simulink model "Target_Control_System"  (R2021b)
settings: Solver=FixedStepDiscrete  StartTime=0.0  StopTime=5  RelTol=1e-3
PreLoadFcn:
  | RTWConfigurationCB('preloadfcn', bdroot);
PostLoadFcn:
  | load('configuration/data_struct.mat');
  | load('configuration/fluxMaps_propMotor.mat');
  | load('configuration/parameterInit_PROP.mat');
  | load('configuration/parameterInit_PUMP.mat');
  | load('configuration/parameterInit_PITCH.mat');
  | load('configuration/parameterInit_TILT.mat');
  | %load('configuration/base_workspace_signal_definition.mat');
  | %load('resolvedatastores_to_baseworkspace_for_faster_simulation.mat');
model workspace (MAT data in the model file):
  SIMULATION_OPTIONS : Simulink.Parameter (value not decoded)
  TARGET_CODE_GEN : Simulink.Parameter (value not decoded)
  TCS_SAMPLE_FREQ_HZ : Simulink.Parameter (value not decoded)
symbols that are objects in the model workspace (value not decoded): TARGET_CODE_GEN, TCS_SAMPLE_FREQ_HZ
undefined symbols (not defined in the file): A_DQ_REF_LPF_INIT__PITCH, A_DQ_REF_LPF_INIT__PROP, A_DQ_REF_LPF_INIT__PUMP, A_DQ_REF_LPF_INIT__TILT, A_OBSERVER_CONFIDENCE_INIT__PITCH, A_OBSERVER_CONFIDENCE_INIT__PROP, A_OBSERVER_CONFIDENCE_INIT__PUMP, A_OBSERVER_CONFIDENCE_INIT__TILT, ACTUATOR_MAX_ANGLE_TRIP__PITCH, ACTUATOR_MIN_ANGLE_TRIP__PITCH, ACTUATOR_POS_SENSOR_INV_DIRECTION__PITCH, ACTUATOR_POS_SENSOR_INV_DIRECTION__TILT, ACTUATOR_POS_SENSOR_OFFSET__PITCH, ACTUATOR_POS_SENSOR_OFFSET__TILT, ADC_scaler1_baseaddr_TILT, ADC_SCALER_FLOAT_TO_FIXPOINT_EXPANSION, ANGLE_ELEC_FROM_SENSOR_OFFSET_INIT__PITCH, ANGLE_ELEC_FROM_SENSOR_OFFSET_INIT__PROP, ANGLE_ELEC_FROM_SENSOR_OFFSET_INIT__PUMP, ANGLE_ELEC_FROM_SENSOR_OFFSET_INIT__TILT, AUTO_CLEAR_FAULTS_ENABLED__PITCH, AUTO_CLEAR_FAULTS_ENABLED__PROP, AUTO_CLEAR_FAULTS_ENABLED__PUMP, AUTO_CLEAR_FAULTS_ENABLED__TILT, AUTO_CLEAR_FAULTS_WAIT_TICKS__PITCH, AUTO_CLEAR_FAULTS_WAIT_TICKS__PROP, AUTO_CLEAR_FAULTS_WAIT_TICKS__PUMP, AUTO_CLEAR_FAULTS_WAIT_TICKS__TILT, AUTO_I_ZERO_IDLE_TICKS__PITCH, AUTO_I_ZERO_IDLE_TICKS__PROP, AUTO_I_ZERO_IDLE_TICKS__PUMP, AUTO_I_ZERO_IDLE_TICKS__TILT, AUTO_I_ZERO_OFFSET_IDC_THRESHOLD__PITCH, AUTO_I_ZERO_OFFSET_IDC_THRESHOLD__PROP, AUTO_I_ZERO_OFFSET_IDC_THRESHOLD__PUMP, AUTO_I_ZERO_OFFSET_IDC_THRESHOLD__TILT, AUTO_I_ZERO_OFFSET_IPH_THRESHOLD__PITCH, AUTO_I_ZERO_OFFSET_IPH_THRESHOLD__PROP, AUTO_I_ZERO_OFFSET_IPH_THRESHOLD__PUMP, AUTO_I_ZERO_OFFSET_IPH_THRESHOLD__TILT, AUTO_SENSORLESS_SWITCHOVER_DISABLE_OMEGA, AUTO_SENSORLESS_SWITCHOVER_ENABLE_OMEGA, AUTO_SENSORLESS_SWITCHOVER_MIN_CONFIDENCE, AUXILIARY_PROTECTION_UNIT_BASEADDR__TILT, blanking_max_error_omega_INIT_PITCH, blanking_max_error_omega_INIT_TILT, blanking_max_error_position_INIT_PITCH, blanking_max_error_position_INIT_TILT, BRUTE_START_I_Q_REF_RAMP_SPEED__PITCH, BRUTE_START_I_Q_REF_RAMP_SPEED__PROP, BRUTE_START_I_Q_REF_RAMP_SPEED__PUMP, BRUTE_START_I_Q_REF_RAMP_SPEED__TILT, CONTROL_LOOP_DT_INIT__PITCH, CONTROL_LOOP_DT_INIT__PROP, CONTROL_LOOP_DT_INIT__PUMP, CONTROL_LOOP_DT_INIT__TILT, CORRECTION_FILTER_SCALE__PITCH, CORRECTION_FILTER_SCALE__PROP, CORRECTION_FILTER_SCALE__PUMP, CORRECTION_FILTER_SCALE__TILT ... (+458)
libraries: simulink x178, Reusables_Lib x24
(part 34 of 47)

== system Target_Control_System/Target_Control_System/MainLoop/pumpMotor_mainLoop/motorTaskMainFastStep(&oPump)/Control Loops - Pump/Sim Options Pump OmegaERef Variant Subsystem/Sim Options 1 Pump OmegaE Subsystem ==
  Constant : Constant  Value=2000  OutDataTypeStr=single  SampleTime=-1
  Constant1 : Constant  Value=0  OutDataTypeStr=uint32  SampleTime=-1
  Data Store Write : DataStoreWrite  DataStoreName=oPump  DataStoreElements=oPump.oMot_.oState_.oRampDataOmegaERef_.fSetpoint_  IndexOptions=Index vector (dialog)  Indices=1  OutputSizes=1
  Data Store Write1 : DataStoreWrite  DataStoreName=oPump  DataStoreElements=oPump.oMot_.oState_.uiSpeedControllerActive_  IndexOptions=Index vector (dialog)  Indices=1  OutputSizes=1
  Out1 : Outport
  wires:
  Constant1/1 -> Data Store Write1/1
  Constant/1 -> Data Store Write/1, Out1/1

== system Target_Control_System/Target_Control_System/MainLoop/pumpMotor_mainLoop/motorTaskMainFastStep(&oPump)/Control Loops - Pump/Subsystem/Set Iq Ref Pump ==
  fIqRefFromSpeedController : Inport
  Enable : EnablePort
  Data Store Read : DataStoreRead  DataStoreName=oPitch  DataStoreElements=oPitch.oMot_.oState_.oFilterDataForSpeedControlIqRef_.afConstantsA_.h0  IndexOptions=Index vector (dialog)  Indices=1  OutputSizes=1
  Data Store Read1 : DataStoreRead  DataStoreName=oPitch  DataStoreElements=oPitch.oMot_.oState_.oFilterDataForSpeedControlIqRef_.afConstantsA_.h1  IndexOptions=Index vector (dialog)  Indices=1  OutputSizes=1
  Data Store Read2 : DataStoreRead  DataStoreName=oPitch  DataStoreElements=oPitch.oMot_.oState_.oFilterDataForSpeedControlIqRef_.afConstantsA_.h2  IndexOptions=Index vector (dialog)  Indices=1  OutputSizes=1
  Data Store Read3 : DataStoreRead  DataStoreName=oPitch  DataStoreElements=oPitch.oMot_.oState_.oFilterDataForSpeedControlIqRef_.afConstantsB_.h0  IndexOptions=Index vector (dialog)  Indices=1  OutputSizes=1
  Data Store Read4 : DataStoreRead  DataStoreName=oPitch  DataStoreElements=oPitch.oMot_.oState_.oFilterDataForSpeedControlIqRef_.afConstantsB_.h1  IndexOptions=Index vector (dialog)  Indices=1  OutputSizes=1
  Data Store Read5 : DataStoreRead  DataStoreName=oPitch  DataStoreElements=oPitch.oMot_.oState_.oFilterDataForSpeedControlIqRef_.afConstantsB_.h2  IndexOptions=Index vector (dialog)  Indices=1  OutputSizes=1
  Data Store Read6 : DataStoreRead  DataStoreName=oPitch  DataStoreElements=oPitch.oMot_.oState_.oFilterDataForSpeedControlIqRef_.afPreviousInputs_.h0  IndexOptions=Index vector (dialog)  Indices=1  OutputSizes=1
  Data Store Read7 : DataStoreRead  DataStoreName=oPitch  DataStoreElements=oPitch.oMot_.oState_.oFilterDataForSpeedControlIqRef_.afPreviousInputs_.h1  IndexOptions=Index vector (dialog)  Indices=1  OutputSizes=1
  Data Store Read8 : DataStoreRead  DataStoreName=oPitch  DataStoreElements=oPitch.oMot_.oState_.oFilterDataForSpeedControlIqRef_.afPreviousOutputs_.h0  IndexOptions=Index vector (dialog)  Indices=1  OutputSizes=1
  Data Store Read9 : DataStoreRead  DataStoreName=oPitch  DataStoreElements=oPitch.oMot_.oState_.oFilterDataForSpeedControlIqRef_.afPreviousOutputs_.h1  IndexOptions=Index vector (dialog)  Indices=1  OutputSizes=1
  Data Store Write1 : DataStoreWrite  DataStoreName=oPitch  DataStoreElements=oPitch.oMot_.oState_.oFilterDataForSpeedControlIqRef_.fFilterOutput_  IndexOptions=Index vector (dialog)  Indices=1  OutputSizes=1
  Data Store Write2 : DataStoreWrite  DataStoreName=oPitch  DataStoreElements=oPitch.oMot_.oState_.oFilterDataForSpeedControlIqRef_.afPreviousOutputs_.h0  IndexOptions=Index vector (dialog)  Indices=1  OutputSizes=1
  Data Store Write3 : DataStoreWrite  DataStoreName=oPitch  DataStoreElements=oPitch.oMot_.oState_.oFilterDataForSpeedControlIqRef_.afPreviousOutputs_.h1  IndexOptions=Index vector (dialog)  Indices=1  OutputSizes=1
  Data Store Write4 : DataStoreWrite  DataStoreName=oPitch  DataStoreElements=oPitch.oMot_.oState_.oFilterDataForSpeedControlIqRef_.afPreviousInputs_.h0  IndexOptions=Index vector (dialog)  Indices=1  OutputSizes=1
  Data Store Write5 : DataStoreWrite  DataStoreName=oPitch  DataStoreElements=oPitch.oMot_.oState_.oFilterDataForSpeedControlIqRef_.afPreviousInputs_.h1  IndexOptions=Index vector (dialog)  Indices=1  OutputSizes=1
  softwareIirFilterStep() : Subsystem
  fIqRefBeforeRamp : Outport
  wires:
  softwareIirFilterStep()/1(*afPreviousInputs1) -> Data Store Write5/1
  softwareIirFilterStep()/2(*afPreviousInputs0) -> Data Store Write4/1
  softwareIirFilterStep()/3(*afPreviousOutputs1) -> Data Store Write3/1
  softwareIirFilterStep()/4(*afPreviousOutputs0) -> Data Store Write2/1
  softwareIirFilterStep()/5(fFilterOutput) -> Data Store Write1/1
  Data Store Read6/1 -> softwareIirFilterStep()/8(afPreviousInputs0)
  Data Store Read7/1 -> softwareIirFilterStep()/9(afPreviousInputs1)
  Data Store Read8/1 -> softwareIirFilterStep()/10(afPreviousOutputs0)
  Data Store Read9/1 -> softwareIirFilterStep()/11(afPreviousOutputs1)
  Data Store Read2/1 -> softwareIirFilterStep()/7(afConstantsA2)
  Data Store Read1/1 -> softwareIirFilterStep()/6(afConstantsA1)
  Data Store Read/1 -> softwareIirFilterStep()/5(afConstantsA0)
  Data Store Read3/1 -> softwareIirFilterStep()/2(afConstantsB0)
  Data Store Read4/1 -> softwareIirFilterStep()/3(afConstantsB1)
  Data Store Read5/1 -> softwareIirFilterStep()/4(afConstantsB2)
  fIqRefFromSpeedController/1 -> softwareIirFilterStep()/1(newInput), fIqRefBeforeRamp/1

== system Target_Control_System/Target_Control_System/MainLoop/pumpMotor_mainLoop/motorTaskMainFastStep(&oPump)/Control Loops - Pump/Subsystem/piControllerStep(&oPiDataRpm_) ==
  fActual : Inport
  fTarget : Inport  Port=2
  fScale : Inport  Port=3
  Enable : EnablePort
  Data Store Read62 : DataStoreRead  DataStoreName=oPump  DataStoreElements=oPump.oMot_.oParam_.oPiDataRpm_.oParameter_.fOutMin_  IndexOptions=Index vector (dialog)  Indices=1  OutputSizes=1
  Data Store Read81 : DataStoreRead  DataStoreName=oPump  DataStoreElements=oPump.oMot_.oParam_.oPiDataRpm_.oParameter_.fKp_  IndexOptions=Index vector (dialog)  Indices=1  OutputSizes=1
  Data Store Read85 : DataStoreRead  DataStoreName=oPump  DataStoreElements=oPump.oMot_.oParam_.oPiDataRpm_.fState_  IndexOptions=Index vector (dialog)  Indices=1  OutputSizes=1
  Data Store Read86 : DataStoreRead  DataStoreName=oPump  DataStoreElements=oPump.oMot_.oParam_.oPiDataRpm_.oParameter_.fLoopDt_  IndexOptions=Index vector (dialog)  Indices=1  OutputSizes=1
  Data Store Read88 : DataStoreRead  DataStoreName=oPump  DataStoreElements=oPump.oMot_.oParam_.oPiDataRpm_.oParameter_.fIntMax_  IndexOptions=Index vector (dialog)  Indices=1  OutputSizes=1
  Data Store Read89 : DataStoreRead  DataStoreName=oPump  DataStoreElements=oPump.oMot_.oParam_.oPiDataRpm_.oParameter_.fOutMax_  IndexOptions=Index vector (dialog)  Indices=1  OutputSizes=1
  Data Store Read90 : DataStoreRead  DataStoreName=oPump  DataStoreElements=oPump.oMot_.oParam_.oPiDataRpm_.oParameter_.fIntMin_  IndexOptions=Index vector (dialog)  Indices=1  OutputSizes=1
  Data Store Read91 : DataStoreRead  DataStoreName=oPump  DataStoreElements=oPump.oMot_.oParam_.oPiDataRpm_.oParameter_.fKi_  IndexOptions=Index vector (dialog)  Indices=1  OutputSizes=1
  Data Store Write21 : DataStoreWrite  DataStoreName=oPump  DataStoreElements=oPump.oMot_.oParam_.oPiDataRpm_.fState_  IndexOptions=Index vector (dialog)  Indices=1  OutputSizes=1
  oPiDataRpm_ : Subsystem
  fOutput : Outport
  wires:
  Data Store Read62/1 -> oPiDataRpm_/10(fOutMin)
  fActual/1 -> oPiDataRpm_/1(fActual)
  fScale/1 -> oPiDataRpm_/5(fScale)
  Data Store Read88/1 -> oPiDataRpm_/7(fIntMax)
  Data Store Read86/1 -> oPiDataRpm_/6(fLoopDt)
  oPiDataRpm_/2(*fpState) -> Data Store Write21/1
  oPiDataRpm_/1(fOutput) -> fOutput/1
  fTarget/1 -> oPiDataRpm_/2(fTarget)
  Data Store Read91/1 -> oPiDataRpm_/4(fKi)
  Data Store Read89/1 -> oPiDataRpm_/8(fOutMax)
  Data Store Read90/1 -> oPiDataRpm_/9(fIntMin)
  Data Store Read85/1 -> oPiDataRpm_/11(fState)
  Data Store Read81/1 -> oPiDataRpm_/3(fKp)

== system Target_Control_System/Target_Control_System/MainLoop/pumpMotor_mainLoop/motorTaskMainFastStep(&oPump)/Control Loops - Pump/Subsystem/pid2ControllerStep(&oPid2DataRpmCtrl_) ==
  fState : Inport
  fActual : Inport  Port=2
  fTarget : Inport  Port=3
  fActualDdt : Inport  Port=4
  Enable : EnablePort
  Data Store Read1 : DataStoreRead  DataStoreName=oPump  DataStoreElements=oPump.oMot_.oParam_.oPid2DataRpmCtrl_.oParameter_.fKi_  IndexOptions=Index vector (dialog)  Indices=1  OutputSizes=1
  Data Store Read10 : DataStoreRead  DataStoreName=oPump  DataStoreElements=oPump.oMot_.oParam_.oPid2DataRpmCtrl_.oParameter_.ipInhibitTarget_  IndexOptions=Index vector (dialog)  Indices=1  OutputSizes=1
  Data Store Read11 : DataStoreRead  DataStoreName=oPump  DataStoreElements=oPump.oMot_.oParam_.oPid2DataRpmCtrl_.oParameter_.fBlankingMaxError_  IndexOptions=Index vector (dialog)  Indices=1  OutputSizes=1
  Data Store Read12 : DataStoreRead  DataStoreName=oPump  DataStoreElements=oPump.oMot_.oParam_.oPid2DataRpmCtrl_.oParameter_.fLargeErrorThresholdNegative_  IndexOptions=Index vector (dialog)  Indices=1  OutputSizes=1
  Data Store Read13 : DataStoreRead  DataStoreName=oPump  DataStoreElements=oPump.oMot_.oParam_.oPid2DataRpmCtrl_.oParameter_.fLargeErrorThresholdPositive_  IndexOptions=Index vector (dialog)  Indices=1  OutputSizes=1
  Data Store Read14 : DataStoreRead  DataStoreName=oPump  DataStoreElements=oPump.oMot_.oParam_.oPid2DataRpmCtrl_.oParameter_.fIntegratorLeakFactor_  IndexOptions=Index vector (dialog)  Indices=1  OutputSizes=1
  Data Store Read15 : DataStoreRead  DataStoreName=oPump  DataStoreElements=oPump.oMot_.oParam_.oPid2DataRpmCtrl_.oParameter_.fErrorReduction_  IndexOptions=Index vector (dialog)  Indices=1  OutputSizes=1
  Data Store Read2 : DataStoreRead  DataStoreName=oPump  DataStoreElements=oPump.oMot_.oParam_.oPid2DataRpmCtrl_.oParameter_.fKd_  IndexOptions=Index vector (dialog)  Indices=1  OutputSizes=1
  Data Store Read20 : DataStoreRead  DataStoreName=oPump  DataStoreElements=oPump.oMot_.oParam_.oPid2DataRpmCtrl_.oParameter_.fKp_  IndexOptions=Index vector (dialog)  Indices=1  OutputSizes=1
  Data Store Read3 : DataStoreRead  DataStoreName=oPump  DataStoreElements=oPump.oMot_.oParam_.oPid2DataRpmCtrl_.oParameter_.fIntMin_  IndexOptions=Index vector (dialog)  Indices=1  OutputSizes=1
  Data Store Read4 : DataStoreRead  DataStoreName=oPump  DataStoreElements=oPump.oMot_.oParam_.oPid2DataRpmCtrl_.oParameter_.fIntMax_  IndexOptions=Index vector (dialog)  Indices=1  OutputSizes=1
  Data Store Read5 : DataStoreRead  DataStoreName=oPump  DataStoreElements=oPump.oMot_.oParam_.oPid2DataRpmCtrl_.oParameter_.fDMin_  IndexOptions=Index vector (dialog)  Indices=1  OutputSizes=1
  Data Store Read6 : DataStoreRead  DataStoreName=oPump  DataStoreElements=oPump.oMot_.oParam_.oPid2DataRpmCtrl_.oParameter_.fDMax_  IndexOptions=Index vector (dialog)  Indices=1  OutputSizes=1
  Data Store Read7 : DataStoreRead  DataStoreName=oPump  DataStoreElements=oPump.oMot_.oParam_.oPid2DataRpmCtrl_.oParameter_.fOutMin_  IndexOptions=Index vector (dialog)  Indices=1  OutputSizes=1
  Data Store Read8 : DataStoreRead  DataStoreName=oPump  DataStoreElements=oPump.oMot_.oParam_.oPid2DataRpmCtrl_.oParameter_.fOutMax_  IndexOptions=Index vector (dialog)  Indices=1  OutputSizes=1
  Data Store Read9 : DataStoreRead  DataStoreName=oPump  DataStoreElements=oPump.oMot_.oParam_.oPid2DataRpmCtrl_.oParameter_.fLoopDt_  IndexOptions=Index vector (dialog)  Indices=1  OutputSizes=1
  Data Store Write5 : DataStoreWrite  DataStoreName=oPump  DataStoreElements=oPump.oMot_.oParam_.oPid2DataRpmCtrl_.fState_  IndexOptions=Index vector (dialog)  Indices=1  OutputSizes=1
  pid2ControllerStep(oPidDataRpmCtrl) : Subsystem  TreatAsAtomicUnit=on
  fOutput : Outport
  wires:
  Data Store Read15/1 -> pid2ControllerStep(oPidDataRpmCtrl)/19(fErrorReduction)
  Data Store Read14/1 -> pid2ControllerStep(oPidDataRpmCtrl)/20(fIntegratorLeakFactor)
  Data Store Read13/1 -> pid2ControllerStep(oPidDataRpmCtrl)/18(fLargeErrorThresholdPositive)
  Data Store Read12/1 -> pid2ControllerStep(oPidDataRpmCtrl)/17(fLargeErrorThresholdNegative)
  Data Store Read11/1 -> pid2ControllerStep(oPidDataRpmCtrl)/16(fBlankingMaxError)
  Data Store Read10/1 -> pid2ControllerStep(oPidDataRpmCtrl)/15(ipInhibitTarget)
  Data Store Read9/1 -> pid2ControllerStep(oPidDataRpmCtrl)/14(fLoopDt)
  Data Store Read8/1 -> pid2ControllerStep(oPidDataRpmCtrl)/13(fOutMax)
  Data Store Read7/1 -> pid2ControllerStep(oPidDataRpmCtrl)/12(fOutMin)
  Data Store Read6/1 -> pid2ControllerStep(oPidDataRpmCtrl)/11(fDMax)
  Data Store Read5/1 -> pid2ControllerStep(oPidDataRpmCtrl)/10(fDMin)
  Data Store Read4/1 -> pid2ControllerStep(oPidDataRpmCtrl)/9(fIntMax)
  Data Store Read3/1 -> pid2ControllerStep(oPidDataRpmCtrl)/8(fIntMin)
  Data Store Read2/1 -> pid2ControllerStep(oPidDataRpmCtrl)/7(fKd)
  Data Store Read1/1 -> pid2ControllerStep(oPidDataRpmCtrl)/6(fKi)
  Data Store Read20/1 -> pid2ControllerStep(oPidDataRpmCtrl)/5(fKp)
  pid2ControllerStep(oPidDataRpmCtrl)/5(fOutput) -> fOutput/1
  pid2ControllerStep(oPidDataRpmCtrl)/6(*fpState) -> Data Store Write5/1
  fActualDdt/1 -> pid2ControllerStep(oPidDataRpmCtrl)/4(fActualDt)
  fState/1 -> pid2ControllerStep(oPidDataRpmCtrl)/3(fpState)
  fTarget/1 -> pid2ControllerStep(oPidDataRpmCtrl)/2(fTarget)
  fActual/1 -> pid2ControllerStep(oPidDataRpmCtrl)/1(fActual)

== system Target_Control_System/Target_Control_System/MainLoop/pumpMotor_mainLoop/motorTaskMainFastStep(&oPump)/Control Loops - Pump/Subsystem2/Subsystem ==
  fFluxWeakeningModulationTarget_ : Inport
  fModulationIndexSquared : Inport  Port=2
  fFluxWeakeningState_ : Inport  Port=3
  fIntControlLoopDt_ : Inport  Port=4
  Enable : EnablePort
  Add : Sum  Inputs=|++
  Add3 : Sum  Inputs=-+
  Constant4 : Constant  Value=0  OutDataTypeStr=single  SampleTime=-1
  Data Store Read94 : DataStoreRead  DataStoreName=oPump  DataStoreElements=oPump.oMot_.oParam_.fFluxWeakeningUpRampGain_  IndexOptions=Index vector (dialog)  Indices=1  OutputSizes=1
  Data Store Read96 : DataStoreRead  DataStoreName=oPump  DataStoreElements=oPump.oMot_.oParam_.fFluxWeakeningMaxCurrent_  IndexOptions=Index vector (dialog)  Indices=1  OutputSizes=1
  Display : Display
  Product : Product
  Product3 : Product
  Saturation Dynamic : simulink/Discontinuities/Saturation Dynamic  OutMin=[]  OutMax=[]  OutDataTypeStr=Inherit: Same as second input  OutDataType=fixdt(1, 16)  OutScaling=2^-10  DoSatur=off
  Out1 : Outport
  wires:
  Constant4/1 -> Saturation Dynamic/3
  Add/1 -> Saturation Dynamic/2
  Product/1 -> Add/1
  Product3/1 -> Product/1
  fIntControlLoopDt_/1 -> Product/2
  fFluxWeakeningState_/1 -> Add/2
  Data Store Read96/1 -> Display/1, Saturation Dynamic/1
  Add3/1 -> Product3/1  "fDelta"
  fFluxWeakeningModulationTarget_/1 -> Add3/1
  fModulationIndexSquared/1 -> Add3/2
  Saturation Dynamic/1 -> Out1/1
  Data Store Read94/1 -> Product3/2

== system Target_Control_System/Target_Control_System/MainLoop/pumpMotor_mainLoop/motorTaskMainFastStep(&oPump)/Control Loops - Pump/Subsystem2/Subsystem1 ==
  fFluxWeakeningDownRamp_ : Inport
  fIntControlLoopDt_ : Inport  Port=2
  fFluxWeakeningState_ : Inport  Port=3
  Enable : EnablePort
  Add13 : Sum  Inputs=-+
  Constant4 : Constant  Value=0  OutDataTypeStr=single  SampleTime=-1
  Product2 : Product
  Switch9 : Switch  Criteria=u2 > Threshold
  Out1 : Outport
  wires:
  Constant4/1 -> Switch9/3
  Add13/1 -> Switch9/1
  Switch9/1 -> Out1/1
  fFluxWeakeningState_/1 -> Add13/2, Switch9/2
  fFluxWeakeningDownRamp_/1 -> Product2/1
  Product2/1 -> Add13/1
  fIntControlLoopDt_/1 -> Product2/2

== system Target_Control_System/Target_Control_System/MainLoop/pumpMotor_mainLoop/motorTaskMainFastStep(&oPump)/Correction Constants for Observer and Control - Pump/Variant Subsystem/Simulation Subsystem IIR Voltage Filter Freq ==
  In1 : Inport
  Gain6 : Gain  Gain=1/(6000*2*pi)
  Out1 : Outport
  wires:
  Gain6/1 -> Out1/1
  In1/1 -> Gain6/1

== system Target_Control_System/Target_Control_System/MainLoop/pumpMotor_mainLoop/motorTaskMainFastStep(&oPump)/Correction Constants for Observer and Control - Pump/Variant Subsystem/Target Code Gen Subsystem IIR Voltage Filter Freq ==
  In1 : Inport
  Data Store Read9 : DataStoreRead  DataStoreName=oPump  DataStoreElements=oPump.oMot_.oParam_.fUphaseIirFLpfRads_  IndexOptions=Index vector (dialog)  Indices=1  OutputSizes=1
  Divide2 : Product  Inputs=*/
  Out1 : Outport
  wires:
  Data Store Read9/1 -> Divide2/2
  In1/1 -> Divide2/1
  Divide2/1 -> Out1/1

== system Target_Control_System/Target_Control_System/MainLoop/pumpMotor_mainLoop/motorTaskMainFastStep(&oPump)/PWM for Simulation/Subsystem1/Subsystem ==
  Enable : EnablePort
  Bus Creator2 : BusCreator  Inputs=3
  Data Store Read2 : DataStoreRead  DataStoreName=oPump  DataStoreElements=oPump.oMot_.oOut_.uiPwmDutyTicksFromMainA_  IndexOptions=Index vector (dialog)  Indices=1  OutputSizes=1
  Data Store Read3 : DataStoreRead  DataStoreName=oPump  DataStoreElements=oPump.oMot_.oOut_.uiPwmDutyTicksFromMainB_  IndexOptions=Index vector (dialog)  Indices=1  OutputSizes=1
  Data Store Read5 : DataStoreRead  DataStoreName=oPump  DataStoreElements=oPump.oMot_.oOut_.uiPwmDutyTicksFromMainC_  IndexOptions=Index vector (dialog)  Indices=1  OutputSizes=1
  pumpMotor_PWMticks : Outport
  wires:
  Data Store Read3/1 -> Bus Creator2/2  "Bticks"
  Data Store Read5/1 -> Bus Creator2/3  "Cticks"
  Bus Creator2/1 -> pumpMotor_PWMticks/1
  Data Store Read2/1 -> Bus Creator2/1  "Aticks"

== system Target_Control_System/Target_Control_System/MainLoop/pumpMotor_mainLoop/motorTaskMainFastStep(&oPump)/Variant Subsystem/Target_Code_Gen_1/Triggered Subsystem ==
  Trigger : TriggerPort  VariantControl=Variant  InitialTriggerSignalState=zero
  Function-Call Generator : simulink/Ports & Subsystems/Function-Call Generator  sample_time=-1  numberOfIterations=1  DisallowWideOutput=off
  Output : Outport
  wires:
  Function-Call Generator/1 -> Output/1

== system Target_Control_System/Target_Control_System/MainLoop/tiltMotor_mainLoop/Decimation gate for 10 Hz Tilt/Function-Call Subsystem/Dynamic_current_limiting/Enabled Subsystem ==
  Enable : EnablePort
  Constant : Constant  Value=0  OutDataTypeStr=single  SampleTime=-1
  Constant1 : Constant  Value=200  OutDataTypeStr=single  SampleTime=-1
  Constant2 : Constant  Value=0  OutDataTypeStr=uint32  SampleTime=-1
  Constant3 : Constant  Value=0  OutDataTypeStr=single  SampleTime=-1
  Constant4 : Constant  Value=0  OutDataTypeStr=uint32  SampleTime=-1
  Data Store Read : DataStoreRead  DataStoreName=oTilt  DataStoreElements=oTilt.oMot_.oParam_.fDynILimDynamicMax_  IndexOptions=Index vector (dialog)  Indices=1  OutputSizes=1
  Data Store Read1 : DataStoreRead  DataStoreName=oTilt  DataStoreElements=oTilt.oMot_.oParam_.fDynILimKnockdownFactor_  IndexOptions=Index vector (dialog)  Indices=1  OutputSizes=1
  Data Store Read3 : DataStoreRead  DataStoreName=oTilt  DataStoreElements=oTilt.oMot_.oState_.fDynILimIntegrator_  IndexOptions=Index vector (dialog)  Indices=1  OutputSizes=1
  Data Store Read4 : DataStoreRead  DataStoreName=oTilt  DataStoreElements=oTilt.oMot_.oParam_.oPiDataRpm_.oParameter_.fOutMin_  IndexOptions=Index vector (dialog)  Indices=1  OutputSizes=1
  Data Store Read5 : DataStoreRead  DataStoreName=oTilt  DataStoreElements=oTilt.oMot_.oState_.fDynILimActualLimit_  IndexOptions=Index vector (dialog)  Indices=1  OutputSizes=1
  Data Store Read6 : DataStoreRead  DataStoreName=oTilt  DataStoreElements=oTilt.oMot_.oParam_.oPiDataRpm_.oParameter_.fIntMin_  IndexOptions=Index vector (dialog)  Indices=1  OutputSizes=1
  Data Store Read7 : DataStoreRead  DataStoreName=oTilt  DataStoreElements=oTilt.oMot_.oState_.uiDriveState_  IndexOptions=Index vector (dialog)  Indices=1  OutputSizes=1
  Data Store Read8 : DataStoreRead  DataStoreName=oTilt  DataStoreElements=oTilt.oMot_.oOut_.uiEnableGateDrive_  IndexOptions=Index vector (dialog)  Indices=1  OutputSizes=1
  Data Store Read9 : DataStoreRead  DataStoreName=oTilt  DataStoreElements=oTilt.oMot_.oOut_.uiCurrentControllerActive_  IndexOptions=Index vector (dialog)  Indices=1  OutputSizes=1
  Data Store Write : DataStoreWrite  DataStoreName=oTilt  DataStoreElements=oTilt.oMot_.oState_.fDynILimIntegrator_  IndexOptions=Index vector (dialog)  Indices=1  OutputSizes=1
  Data Store Write1 : DataStoreWrite  DataStoreName=oTilt  DataStoreElements=oTilt.oMot_.oParam_.oPiDataRpm_.oParameter_.fOutMax_  IndexOptions=Index vector (dialog)  Indices=1  OutputSizes=1
  Data Store Write2 : DataStoreWrite  DataStoreName=oTilt  DataStoreElements=oTilt.oMot_.oParam_.oPiDataRpm_.oParameter_.fOutMin_  IndexOptions=Index vector (dialog)  Indices=1  OutputSizes=1
  Data Store Write3 : DataStoreWrite  DataStoreName=oTilt  DataStoreElements=oTilt.oMot_.oParam_.oPiDataRpm_.oParameter_.fIntMin_  IndexOptions=Index vector (dialog)  Indices=1  OutputSizes=1
  Data Store Write4 : DataStoreWrite  DataStoreName=oTilt  DataStoreElements=oTilt.oMot_.oParam_.oPiDataRpm_.oParameter_.fIntMax_  IndexOptions=Index vector (dialog)  Indices=1  OutputSizes=1
  Data Store Write5 : DataStoreWrite  DataStoreName=oTilt  DataStoreElements=oTilt.oMot_.oOut_.uiEnableGateDrive_  IndexOptions=Index vector (dialog)  Indices=1  OutputSizes=1
  Data Store Write6 : DataStoreWrite  DataStoreName=oTilt  DataStoreElements=oTilt.oMot_.oOut_.uiCurrentControllerActive_  IndexOptions=Index vector (dialog)  Indices=1  OutputSizes=1
  Divide : Product  Inputs=*/
  Gain : Gain  Gain=3
  IsNaN : RelationalOperator  Operator=isNaN  OutDataTypeStr=boolean  RndMeth=Simplest
  Less Than : RelationalOperator  Operator=<  OutDataTypeStr=boolean  RndMeth=Simplest
  Saturation Dynamic : simulink/Discontinuities/Saturation Dynamic  OutMin=[]  OutMax=[]  OutDataTypeStr=Inherit: Same as second input  OutDataType=fixdt(1, 16)  OutScaling=2^-10  DoSatur=off
  Switch{,2..5} (5 alike) : Switch  Criteria=u2 > Threshold
  Unary Minus : UnaryMinus
  Unary Minus1 : UnaryMinus
  wires:
  Unary Minus/1 -> Switch2/1
  Data Store Read3/1 -> IsNaN/1, Switch/3
  Data Store Read5/1 -> Data Store Write4/1, Unary Minus1/1
  Constant4/1 -> Switch5/1
  Gain/1 -> Saturation Dynamic/1
  Constant1/1 -> Less Than/2
  Constant3/1 -> Saturation Dynamic/3
  Data Store Read8/1 -> Switch4/3
  Switch3/1 -> Data Store Write3/1
  Data Store Read9/1 -> Switch5/3
  Switch2/1 -> Data Store Write2/1
  Unary Minus1/1 -> Switch3/1
  Constant2/1 -> Switch4/1
  Less Than/1 -> Switch4/2, Switch5/2
  Switch5/1 -> Data Store Write6/1
  Data Store Read/1 -> Divide/1, Unary Minus/1, Data Store Write1/1
  Data Store Read4/1 -> Switch2/3, Switch2/2
  Data Store Read7/1 -> Less Than/1
  Divide/1 -> Gain/1
  Data Store Read1/1 -> Divide/2
  Saturation Dynamic/1 -> Data Store Write/1  "fDynLimIntegrator"
  IsNaN/1 -> Switch/2
  Switch4/1 -> Data Store Write5/1
  Switch/1 -> Saturation Dynamic/2
  Data Store Read6/1 -> Switch3/3, Switch3/2
  Constant/1 -> Switch/1

== system Target_Control_System/Target_Control_System/MainLoop/tiltMotor_mainLoop/Decimation gate for 200 Hz Tilt/motorTaskMainDecimationAStep(&oTilt)/Check zero current if inverter off/Enabled Subsystem ==
  note: The inverter is idle (mosfets are off), and the current sensors have been offset corrected.
      | The current sensor readings should be fairly close to zero.
  Enable : EnablePort
  Chart : Stateflow chart  TreatAsAtomicUnit=on

== system Target_Control_System/Target_Control_System/MainLoop/tiltMotor_mainLoop/Decimation gate for 200 Hz Tilt/motorTaskMainDecimationAStep(&oTilt)/Current control inactive/Enabled Subsystem ==
  note: Keep the speed controller integrator value at zero
  Enable : EnablePort
  Constant : Constant  Value=0  OutDataTypeStr=single  SampleTime=-1
  Data Store Write : DataStoreWrite  DataStoreName=oTilt  DataStoreElements=oTilt.oMot_.oParam_.oPiDataRpm_.fState_  IndexOptions=Index vector (dialog)  Indices=1  OutputSizes=1
  Data Store Write1 : DataStoreWrite  DataStoreName=oTilt  DataStoreElements=oTilt.oMot_.oParam_.oPid2DataRpmCtrl_.fState_  IndexOptions=Index vector (dialog)  Indices=1  OutputSizes=1
  wires:
  Constant/1 -> Data Store Write/1, Data Store Write1/1

== system Target_Control_System/Target_Control_System/MainLoop/tiltMotor_mainLoop/Decimation gate for 200 Hz Tilt/motorTaskMainDecimationAStep(&oTilt)/Current offset nulling/initiateOffsetNulling(&oTilt) ==
  note: Further checks for starting the nulling process are handled inside the lower level function
  Enable : EnablePort
  Chart : Stateflow chart  TreatAsAtomicUnit=on

== system Target_Control_System/Target_Control_System/MainLoop/tiltMotor_mainLoop/Decimation gate for 200 Hz Tilt/motorTaskMainDecimationAStep(&oTilt)/Forced current injection for broken input sensors/Enabled Subsystem ==
  note: Forced current injection for broken input position sensors:
      | 226 = a signaling state, the inverter is not actually on
      | 227 = the actual on state, pure 0 RPM
      | 228 = rudimentary position control using only the output position sensor
  Enable : EnablePort
  Constant : Constant  OutDataTypeStr=uint32  SampleTime=-1
  Constant1 : Constant  Value=0  OutDataTypeStr=uint32  SampleTime=-1
  Constant2 : Constant  Value=0  OutDataTypeStr=int32  SampleTime=-1
  Constant3 : Constant  Value=228  OutDataTypeStr=uint32  SampleTime=-1
  Data Store Read7 : DataStoreRead  DataStoreName=oTilt  DataStoreElements=oTilt.oMot_.oState_.uiDriveState_  IndexOptions=Index vector (dialog)  Indices=1  OutputSizes=1
  Data Store Write3 : DataStoreWrite  DataStoreName=oTilt  DataStoreElements=oTilt.oMot_.oOut_.uiForcedAngle_  IndexOptions=Index vector (dialog)  Indices=1  OutputSizes=1
  Data Store Write4 : DataStoreWrite  DataStoreName=oTilt  DataStoreElements=oTilt.oMot_.oState_.uiSpeedControllerActive_  IndexOptions=Index vector (dialog)  Indices=1  OutputSizes=1
  Data Store Write5 : DataStoreWrite  DataStoreName=oTilt  DataStoreElements=oTilt.oMot_.oState_.oPosSensor_.iPosControlEnabled_  IndexOptions=Index vector (dialog)  Indices=1  OutputSizes=1
  NOT : Logic  Operator=NOT  IconShape=distinctive  AllPortsSameDT=off  OutDataTypeStr=boolean
  NotEqual : RelationalOperator  Operator=~=  OutDataTypeStr=boolean  RndMeth=Simplest
  Pure_0rpm_holding_mode : Subsystem  TreatAsAtomicUnit=on
  Rudimentary_forced_angle_position_control : Subsystem  TreatAsAtomicUnit=on
  wires:
  Constant2/1 -> Data Store Write5/1
  Constant1/1 -> Data Store Write4/1
  Constant/1 -> Data Store Write3/1
  NOT/1 -> Rudimentary_forced_angle_position_control/Enable
  NotEqual/1 -> Pure_0rpm_holding_mode/Enable, NOT/1
  Constant3/1 -> NotEqual/2
  Data Store Read7/1 -> NotEqual/1

== system Target_Control_System/Target_Control_System/MainLoop/tiltMotor_mainLoop/Decimation gate for 200 Hz Tilt/motorTaskMainDecimationAStep(&oTilt)/Idle controller/Forced angle ==
  Enable : EnablePort
  Data Store Write1 : DataStoreWrite  DataStoreName=oTilt  DataStoreElements=oTilt.oMot_.oState_.fIdleCtrlCurrent_  IndexOptions=Index vector (dialog)  Indices=1  OutputSizes=1
  Data Store Write2 : DataStoreWrite  DataStoreName=oTilt  DataStoreElements=oTilt.oMot_.oParam_.oPiDataIdleCtrl_.fState_  IndexOptions=Index vector (dialog)  Indices=1  OutputSizes=1
  Zero16 : Constant  Value=0  OutDataTypeStr=single  SampleTime=-1
  wires:
  Zero16/1 -> Data Store Write1/1, Data Store Write2/1

== system Target_Control_System/Target_Control_System/MainLoop/tiltMotor_mainLoop/Decimation gate for 200 Hz Tilt/motorTaskMainDecimationAStep(&oTilt)/Idle controller/Not forced angle ==
  Enable : EnablePort
  Data Store Read10 : DataStoreRead  DataStoreName=oTilt  DataStoreElements=oTilt.oMot_.oParam_.oPiDataIdleCtrl_.oParameter_.fIntMax_  IndexOptions=Index vector (dialog)  Indices=1  OutputSizes=1
  Data Store Read11 : DataStoreRead  DataStoreName=oTilt  DataStoreElements=oTilt.oMot_.oParam_.oPiDataIdleCtrl_.oParameter_.fOutMax_  IndexOptions=Index vector (dialog)  Indices=1  OutputSizes=1
  Data Store Read12 : DataStoreRead  DataStoreName=oTilt  DataStoreElements=oTilt.oMot_.oParam_.oPiDataIdleCtrl_.oParameter_.fLoopDt_  IndexOptions=Index vector (dialog)  Indices=1  OutputSizes=1
  Data Store Read13 : DataStoreRead  DataStoreName=oTilt  DataStoreElements=oTilt.oMot_.oParam_.oPiDataIdleCtrl_.fState_  IndexOptions=Index vector (dialog)  Indices=1  OutputSizes=1
  Data Store Read4 : DataStoreRead  DataStoreName=oTilt  DataStoreElements=oTilt.oMot_.oParam_.oPiDataIdleCtrl_.oParameter_.fIntMin_  IndexOptions=Index vector (dialog)  Indices=1  OutputSizes=1
  Data Store Read5 : DataStoreRead  DataStoreName=oTilt  DataStoreElements=oTilt.oMot_.oParam_.oPiDataIdleCtrl_.oParameter_.fOutMin_  IndexOptions=Index vector (dialog)  Indices=1  OutputSizes=1
  Data Store Read6 : DataStoreRead  DataStoreName=oTilt  DataStoreElements=oTilt.oMot_.oOut_.fOmegaEObserverXlpf2_  IndexOptions=Index vector (dialog)  Indices=1  OutputSizes=1
  Data Store Read7 : DataStoreRead  DataStoreName=oTilt  DataStoreElements=oTilt.oMot_.oState_.fIdleCtrlOmegaEMin_  IndexOptions=Index vector (dialog)  Indices=1  OutputSizes=1
  Data Store Read8 : DataStoreRead  DataStoreName=oTilt  DataStoreElements=oTilt.oMot_.oParam_.oPiDataIdleCtrl_.oParameter_.fKp_  IndexOptions=Index vector (dialog)  Indices=1  OutputSizes=1
  Data Store Read9 : DataStoreRead  DataStoreName=oTilt  DataStoreElements=oTilt.oMot_.oParam_.oPiDataIdleCtrl_.oParameter_.fKi_  IndexOptions=Index vector (dialog)  Indices=1  OutputSizes=1
  Data Store Write : DataStoreWrite  DataStoreName=oTilt  DataStoreElements=oTilt.oMot_.oParam_.oPiDataIdleCtrl_.fState_  IndexOptions=Index vector (dialog)  Indices=1  OutputSizes=1
  Data Store Write11 : DataStoreWrite  DataStoreName=oTilt  DataStoreElements=oTilt.oMot_.oState_.fIdleCtrlCurrent_  IndexOptions=Index vector (dialog)  Indices=1  OutputSizes=1
  Zero19 : Constant  OutDataTypeStr=single  SampleTime=-1
  piControllerStep_Idle_Controller(&oTilt) : Subsystem  SystemSampleTime=1/200
  wires:
  Data Store Read6/1 -> piControllerStep_Idle_Controller(&oTilt)/1(fActual)
  Data Store Read7/1 -> piControllerStep_Idle_Controller(&oTilt)/2(fTarget)
  Data Store Read8/1 -> piControllerStep_Idle_Controller(&oTilt)/3(fKp)
  Data Store Read9/1 -> piControllerStep_Idle_Controller(&oTilt)/4(fKi)
  Data Store Read12/1 -> piControllerStep_Idle_Controller(&oTilt)/6(fLoopDt)
  Data Store Read10/1 -> piControllerStep_Idle_Controller(&oTilt)/7(fIntMax)
  Data Store Read11/1 -> piControllerStep_Idle_Controller(&oTilt)/8(fOutMax)
  Data Store Read4/1 -> piControllerStep_Idle_Controller(&oTilt)/9(fIntMin)
  Data Store Read5/1 -> piControllerStep_Idle_Controller(&oTilt)/10(fOutMin)
  piControllerStep_Idle_Controller(&oTilt)/2(*fpState) -> Data Store Write/1
  piControllerStep_Idle_Controller(&oTilt)/1(fOutput) -> Data Store Write11/1

== system Target_Control_System/Target_Control_System/MainLoop/tiltMotor_mainLoop/Decimation gate for 200 Hz Tilt/motorTaskMainDecimationAStep(&oTilt)/Position control checks/NOT position control mode ==
  note: Not in position control mode, so either torque or speed mode (=prop and pumpfan)
      | Evaluate need for blanking (with hysteresis if the confidence is inbetween):
  Enable : EnablePort
  Chart : Stateflow chart  TreatAsAtomicUnit=on

== system Target_Control_System/Target_Control_System/MainLoop/tiltMotor_mainLoop/Decimation gate for 200 Hz Tilt/motorTaskMainDecimationAStep(&oTilt)/Position control checks/Position control mode ==
  Enable : EnablePort
  Check AD2S1210 : Subsystem  Commented=on  TreatAsAtomicUnit=on
  Check fighting controllers : Subsystem  TreatAsAtomicUnit=on
  Check for position halted : Subsystem  TreatAsAtomicUnit=on
  Function-Call Generator : simulink/Ports & Subsystems/Function-Call Generator  sample_time=-1  numberOfIterations=1  DisallowWideOutput=off
  Function-Call Split1 : FunctionCallSplit  NumOutputPorts=2
  Function-Call Split10 : FunctionCallSplit  NumOutputPorts=2
  Function-Call Split2 : FunctionCallSplit  NumOutputPorts=2
  checkSensorLimits(&oTilt) : Subsystem  TreatAsAtomicUnit=on
  wires:
  Function-Call Split2/2 -> Check fighting controllers/Trigger
  Function-Call Split2/1 -> Check AD2S1210/Trigger
  Function-Call Split1/2 -> Function-Call Split2/1
  Function-Call Split1/1 -> checkSensorLimits(&oTilt)/Trigger
  Function-Call Split10/2 -> Function-Call Split1/1
  Function-Call Split10/1 -> Check for position halted/Trigger
  Function-Call Generator/1 -> Function-Call Split10/1

== system Target_Control_System/Target_Control_System/MainLoop/tiltMotor_mainLoop/Decimation gate for 5000 Hz Tilt/motorTaskProcessExternalSetpoints(&oTilt)/hot_standby/Subsystem ==
  Enable : EnablePort
  Data Store Write19 : DataStoreWrite  DataStoreName=oTilt  DataStoreElements=oTilt.oMot_.oIn_.fIqSetpoint_  IndexOptions=Index vector (dialog)  Indices=1  OutputSizes=1
  const : Constant  Value=0.0  OutDataTypeStr=single  SampleTime=-1
  wires:
  const/1 -> Data Store Write19/1

== system Target_Control_System/Target_Control_System/MainLoop/tiltMotor_mainLoop/Decimation gate for 5000 Hz Tilt/motorTaskProcessExternalSetpoints(&oTilt)/passive_holding_mode/Subsystem ==
  Enable : EnablePort
  Data Store Read68 : DataStoreRead  DataStoreName=oTilt  DataStoreElements=oTilt.oMot_.oParam_.fDynILimDynamicMax_  IndexOptions=Index vector (dialog)  Indices=1  OutputSizes=1
  Data Store Write19 : DataStoreWrite  DataStoreName=oTilt  DataStoreElements=oTilt.oMot_.oIn_.fIqSetpoint_  IndexOptions=Index vector (dialog)  Indices=1  OutputSizes=1
  wires:
  Data Store Read68/1 -> Data Store Write19/1

== system Target_Control_System/Target_Control_System/MainLoop/tiltMotor_mainLoop/Decimation gate for 5000 Hz Tilt/motorTaskProcessExternalSetpoints(&oTilt)/set_target/Id_target ==
  Enable : EnablePort
  AND1 : Logic  Operator=OR  AllPortsSameDT=off  OutDataTypeStr=boolean
  Data Store Read1 : DataStoreRead  DataStoreName=oTilt  DataStoreElements=oTilt.oMot_.oIn_.fIdSetpoint_  IndexOptions=Index vector (dialog)  Indices=1  OutputSizes=1
  IsNaN : RelationalOperator  Operator=isNaN  OutDataTypeStr=boolean  RndMeth=Simplest
  IsNaN1 : RelationalOperator  Operator=isInf  OutDataTypeStr=boolean  RndMeth=Simplest
  NOT1 : Logic  Operator=NOT  AllPortsSameDT=off  OutDataTypeStr=boolean
  Subsystem : Subsystem
  wires:
  NOT1/1 -> AND1/1
  Data Store Read1/1 -> IsNaN1/1, Subsystem/1(Input), IsNaN/1
  IsNaN1/1 -> AND1/2
  IsNaN/1 -> NOT1/1
  AND1/1 -> Subsystem/Enable

== system Target_Control_System/Target_Control_System/MainLoop/tiltMotor_mainLoop/Decimation gate for 5000 Hz Tilt/motorTaskProcessExternalSetpoints(&oTilt)/set_target/Id_zero_for_forced_angle ==
  Enable : EnablePort
  Data Store Write1 : DataStoreWrite  DataStoreName=oTilt  DataStoreElements=oTilt.oMot_.oState_.fIdExternalSetpoint_  IndexOptions=Index vector (dialog)  Indices=1  OutputSizes=1
  Data Store Write19 : DataStoreWrite  DataStoreName=oTilt  DataStoreElements=oTilt.oMot_.oState_.oRampDataIdRef_.fSetpoint_  IndexOptions=Index vector (dialog)  Indices=1  OutputSizes=1
  const1 : Constant  Value=0.0  OutDataTypeStr=single  SampleTime=-1
  wires:
  const1/1 -> Data Store Write19/1, Data Store Write1/1

== system Target_Control_System/Target_Control_System/MainLoop/tiltMotor_mainLoop/Decimation gate for 5000 Hz Tilt/motorTaskProcessExternalSetpoints(&oTilt)/set_target/Iq_target ==
  Enable : EnablePort
  AND : Logic  AllPortsSameDT=off  OutDataTypeStr=boolean
  AND1 : Logic  AllPortsSameDT=off  OutDataTypeStr=boolean
  Data Store Read1 : DataStoreRead  DataStoreName=oTilt  DataStoreElements=oTilt.oMot_.oState_.uiSpeedControllerActive_  IndexOptions=Index vector (dialog)  Indices=1  OutputSizes=1
  Data Store Read2 : DataStoreRead  DataStoreName=oTilt  DataStoreElements=oTilt.oMot_.oState_.oPosSensor_.iPosControlEnabled_  IndexOptions=Index vector (dialog)  Indices=1  OutputSizes=1
  Data Store Read68 : DataStoreRead  DataStoreName=oTilt  DataStoreElements=oTilt.oMot_.oIn_.fIqSetpoint_  IndexOptions=Index vector (dialog)  Indices=1  OutputSizes=1
  Data Store Read85 : DataStoreRead  DataStoreName=oTilt  DataStoreElements=oTilt.oMot_.oParam_.uiTorqueMirroringActive_  IndexOptions=Index vector (dialog)  Indices=1  OutputSizes=1
  IsNaN : RelationalOperator  Operator=isNaN  OutDataTypeStr=boolean  RndMeth=Simplest
  NOT : Logic  Operator=NOT  AllPortsSameDT=off  OutDataTypeStr=boolean
  NOT1 : Logic  Operator=NOT  AllPortsSameDT=off  OutDataTypeStr=boolean
  NOT2 : Logic  Operator=NOT  AllPortsSameDT=off  OutDataTypeStr=boolean
  OR : Logic  Operator=OR  AllPortsSameDT=off  OutDataTypeStr=boolean
  Subsystem : Subsystem
  wires:
  AND1/1 -> Subsystem/Enable
  Data Store Read85/1 -> OR/1
  Data Store Read1/1 -> NOT/1
  AND/1 -> OR/2
  NOT/1 -> AND/1
  Data Store Read2/1 -> NOT1/1
  NOT1/1 -> AND/2
  OR/1 -> AND1/1
  Data Store Read68/1 -> IsNaN/1
  IsNaN/1 -> NOT2/1
  NOT2/1 -> AND1/2

== system Target_Control_System/Target_Control_System/MainLoop/tiltMotor_mainLoop/Decimation gate for 5000 Hz Tilt/motorTaskProcessExternalSetpoints(&oTilt)/set_target/position_target ==
  Enable : EnablePort
  AND : Logic  Operator=OR  AllPortsSameDT=off  OutDataTypeStr=boolean
  AND1 : Logic  Inputs=3  AllPortsSameDT=off  OutDataTypeStr=boolean
  Data Store Read1 : DataStoreRead  DataStoreName=oTilt  DataStoreElements=oTilt.oMot_.oState_.oPosSensor_.iPosControlEnabled_  IndexOptions=Index vector (dialog)  Indices=1  OutputSizes=1
  Data Store Read68 : DataStoreRead  DataStoreName=oTilt  DataStoreElements=oTilt.oMot_.oIn_.fPosSetpoint_  IndexOptions=Index vector (dialog)  Indices=1  OutputSizes=1
  Data Store Read85 : DataStoreRead  DataStoreName=oTilt  DataStoreElements=oTilt.oMot_.oState_.uiDriveState_  IndexOptions=Index vector (dialog)  Indices=1  OutputSizes=1
  Equal1 : RelationalOperator  Operator=~=  OutDataTypeStr=boolean  RndMeth=Simplest
  Equal13 : RelationalOperator  Operator===  OutDataTypeStr=boolean  RndMeth=Simplest
  IsNaN : RelationalOperator  Operator=isNaN  OutDataTypeStr=boolean  RndMeth=Simplest
  NOT2 : Logic  Operator=NOT  AllPortsSameDT=off  OutDataTypeStr=boolean
  Subsystem : Subsystem
  const1 : Constant  Value=202  OutDataTypeStr=uint32  SampleTime=-1
  const17 : Constant  Value=228  OutDataTypeStr=uint32  SampleTime=-1
  wires:
  NOT2/1 -> AND1/3
  const1/1 -> Equal1/2
  Equal1/1 -> AND1/2
  const17/1 -> Equal13/1
  Data Store Read85/1 -> Equal1/1, Equal13/2
  Equal13/1 -> AND/2
  AND/1 -> AND1/1
  Data Store Read1/1 -> AND/1
  IsNaN/1 -> NOT2/1
  Data Store Read68/1 -> IsNaN/1
  AND1/1 -> Subsystem/Enable

== system Target_Control_System/Target_Control_System/MainLoop/tiltMotor_mainLoop/Decimation gate for 5000 Hz Tilt/motorTaskProcessExternalSetpoints(&oTilt)/set_target/speed_target ==
  Enable : EnablePort
  AND1 : Logic  Inputs=3  AllPortsSameDT=off  OutDataTypeStr=boolean
  Data Store Read1 : DataStoreRead  DataStoreName=oTilt  DataStoreElements=oTilt.oMot_.oState_.oPosSensor_.iPosControlEnabled_  IndexOptions=Index vector (dialog)  Indices=1  OutputSizes=1
  Data Store Read2 : DataStoreRead  DataStoreName=oTilt  DataStoreElements=oTilt.oMot_.oParam_.uiAutomaticFanControlMode_  IndexOptions=Index vector (dialog)  Indices=1  OutputSizes=1
  Data Store Read85 : DataStoreRead  DataStoreName=oTilt  DataStoreElements=oTilt.oMot_.oState_.uiDriveState_  IndexOptions=Index vector (dialog)  Indices=1  OutputSizes=1
  Equal13 : RelationalOperator  Operator=~=  OutDataTypeStr=boolean  RndMeth=Simplest
  NOT1 : Logic  Operator=NOT  AllPortsSameDT=off  OutDataTypeStr=boolean
  NOT2 : Logic  Operator=NOT  AllPortsSameDT=off  OutDataTypeStr=boolean
  Subsystem : Subsystem
  const17 : Constant  Value=228  OutDataTypeStr=uint32  SampleTime=-1
  wires:
  Data Store Read2/1 -> NOT2/1
  NOT2/1 -> AND1/2
  const17/1 -> Equal13/1
  Data Store Read85/1 -> Equal13/2
  Equal13/1 -> AND1/3
  NOT1/1 -> AND1/1
  Data Store Read1/1 -> NOT1/1
  AND1/1 -> Subsystem/Enable

== system Target_Control_System/Target_Control_System/MainLoop/tiltMotor_mainLoop/mainTask_tilt/PWM for Simulation/Subsystem1/Subsystem ==
  Enable : EnablePort
  Bus Creator2 : BusCreator  Inputs=3
  Data Store Read2 : DataStoreRead  DataStoreName=oTilt  DataStoreElements=oTilt.oMot_.oOut_.uiPwmDutyTicksFromMainA_  IndexOptions=Index vector (dialog)  Indices=1  OutputSizes=1
  Data Store Read3 : DataStoreRead  DataStoreName=oTilt  DataStoreElements=oTilt.oMot_.oOut_.uiPwmDutyTicksFromMainB_  IndexOptions=Index vector (dialog)  Indices=1  OutputSizes=1
  Data Store Read5 : DataStoreRead  DataStoreName=oTilt  DataStoreElements=oTilt.oMot_.oOut_.uiPwmDutyTicksFromMainC_  IndexOptions=Index vector (dialog)  Indices=1  OutputSizes=1
  tiltMotor_PWMticks : Outport
  wires:
  Data Store Read3/1 -> Bus Creator2/2  "Bticks"
  Data Store Read5/1 -> Bus Creator2/3  "Cticks"
  Bus Creator2/1 -> tiltMotor_PWMticks/1
  Data Store Read2/1 -> Bus Creator2/1  "Aticks"

== system Target_Control_System/Target_Control_System/MainLoop/tiltMotor_mainLoop/mainTask_tilt/Variant Subsystem/Target_Code_Gen_1/Triggered Subsystem ==
  Trigger : TriggerPort  VariantControl=Variant  InitialTriggerSignalState=zero
  Function-Call Generator : simulink/Ports & Subsystems/Function-Call Generator  sample_time=-1  numberOfIterations=1  DisallowWideOutput=off
  Output : Outport
  wires:
  Function-Call Generator/1 -> Output/1

== system Target_Control_System/Target_Control_System/MainLoop/tiltMotor_mainLoop/mainTask_tilt/motorTaskMainFastStep(&oTilt)/Automatic switching to sensorless - Tilt/Automatic switching to sensorless ==
  note: // Presently disabled, do we need to enable?
  Enable : EnablePort
  Data Store Read1 : DataStoreRead  DataStoreName=oTilt  DataStoreElements=oTilt.oMot_.oState_.uiSensorlessSwitchoverState_  IndexOptions=Index vector (dialog)  Indices=1  OutputSizes=1
  Data Store Read2 : DataStoreRead  DataStoreName=oTilt  DataStoreElements=oTilt.oMot_.oState_.fObserverConfidence_  IndexOptions=Index vector (dialog)  Indices=1  OutputSizes=1
  If : If
  "Switch to sensored " : Subsystem  TreatAsAtomicUnit=on
  Switch to sensorless? : Subsystem  TreatAsAtomicUnit=on
  wires:
  Data Store Read2/1 -> "Switch to sensored "/1(fObserverConfidence), Switch to sensorless?/1(fObserverConfidence)
  Data Store Read1/1 -> If/1
  If/1 -> "Switch to sensored "/Action
  If/2 -> Switch to sensorless?/Action

== system Target_Control_System/Target_Control_System/MainLoop/tiltMotor_mainLoop/mainTask_tilt/motorTaskMainFastStep(&oTilt)/Control Loops - Tilt/Dynamic Current Limiting Tilt ==
  Enable : EnablePort
  Abs : Abs
  Add : Sum  Inputs=+-
  Add1 : Sum
  Add2 : Sum  Inputs=-+
  Data Store Read : DataStoreRead  DataStoreName=oTilt  DataStoreElements=oTilt.oMot_.oIn_.fIPhaseMagnitude_  IndexOptions=Index vector (dialog)  Indices=1  OutputSizes=1
  Data Store Read1 : DataStoreRead  DataStoreName=oTilt  DataStoreElements=oTilt.oMot_.oParam_.fIqSetpointMax_  IndexOptions=Index vector (dialog)  Indices=1  OutputSizes=1
  Data Store Read10 : DataStoreRead  DataStoreName=oTilt  DataStoreElements=oTilt.oMot_.oParam_.fDynILimIntegratorLeakageFactor_  IndexOptions=Index vector (dialog)  Indices=1  OutputSizes=1
  Data Store Read2 : DataStoreRead  DataStoreName=oTilt  DataStoreElements=oTilt.oMot_.oState_.fDynILimIntegrator_  IndexOptions=Index vector (dialog)  Indices=1  OutputSizes=1
  Data Store Read3 : DataStoreRead  DataStoreName=oTilt  DataStoreElements=oTilt.oMot_.oParam_.fDynILimDynamicMax_  IndexOptions=Index vector (dialog)  Indices=1  OutputSizes=1
  Data Store Read4 : DataStoreRead  DataStoreName=oTilt  DataStoreElements=oTilt.oMot_.oParam_.fTorqueAuthorityFraction_  IndexOptions=Index vector (dialog)  Indices=1  OutputSizes=1
  Data Store Read5 : DataStoreRead  DataStoreName=oTilt  DataStoreElements=oTilt.oMot_.oParam_.fDynILimKnockdownFactor_  IndexOptions=Index vector (dialog)  Indices=1  OutputSizes=1
  Data Store Read6 : DataStoreRead  DataStoreName=oTilt  DataStoreElements=oTilt.oMot_.oState_.fIqRefBeforeRamp_  IndexOptions=Index vector (dialog)  Indices=1  OutputSizes=1
  Data Store Read7 : DataStoreRead  DataStoreName=oTilt  DataStoreElements=oTilt.oMot_.oParam_.fDynILimDynamicMax_  IndexOptions=Index vector (dialog)  Indices=1  OutputSizes=1
  Data Store Write : DataStoreWrite  DataStoreName=oTilt  DataStoreElements=oTilt.oMot_.oState_.fDynILimIntegrator_  IndexOptions=Index vector (dialog)  Indices=1  OutputSizes=1
  Data Store Write1 : DataStoreWrite  DataStoreName=oTilt  DataStoreElements=oTilt.oMot_.oState_.fDynILimActualLimit_  IndexOptions=Index vector (dialog)  Indices=1  OutputSizes=1
  Data Store Write3 : DataStoreWrite  DataStoreName=oTilt  DataStoreElements=oTilt.oMot_.oParam_.oPid2DataRpmCtrl_.oParameter_.fOutMax_  IndexOptions=Index vector (dialog)  Indices=1  OutputSizes=1
  Data Store Write4 : DataStoreWrite  DataStoreName=oTilt  DataStoreElements=oTilt.oMot_.oParam_.oPid2DataRpmCtrl_.oParameter_.fOutMin_  IndexOptions=Index vector (dialog)  Indices=1  OutputSizes=1
  Data Store Write5 : DataStoreWrite  DataStoreName=oTilt  DataStoreElements=oTilt.oMot_.oParam_.oPid2DataRpmCtrl_.oParameter_.fIntMin_  IndexOptions=Index vector (dialog)  Indices=1  OutputSizes=1
  Data Store Write6 : DataStoreWrite  DataStoreName=oTilt  DataStoreElements=oTilt.oMot_.oParam_.oPid2DataRpmCtrl_.oParameter_.fIntMax_  IndexOptions=Index vector (dialog)  Indices=1  OutputSizes=1
  Divide{,1..3} (4 alike) : Product  Inputs=**
  Gain : Gain  Gain=-1
  Gain1 : Gain  Gain=-1
  Gain2 : Gain  Gain=-1
  Max : MinMax  Function=max  Inputs=2
  Max1 : MinMax  Function=max  Inputs=2
  Min : MinMax  Inputs=2
  Switch : Switch  Criteria=u2 > Threshold
  oRampDataIqRef_.fSetpoint : Outport
  wires:
  Gain2/1 -> Data Store Write4/1
  Data Store Read7/1 -> Gain2/1, Data Store Write3/1
  Gain1/1 -> Data Store Write5/1
  Max1/1 -> oRampDataIqRef_.fSetpoint/1
  Gain/1 -> Max1/1
  Min/1 -> Max1/2
  Data Store Read6/1 -> Min/2
  Max/1 -> Min/1, Data Store Write1/1, Gain1/1, Data Store Write6/1, Gain/1
  Add2/1 -> Max/1
  Divide2/1 -> Add2/2
  Divide3/1 -> Add2/1
  Data Store Read5/1 -> Divide3/2
  Data Store Read4/1 -> Divide2/2
  Data Store Read3/1 -> Divide2/1
  Divide1/1 -> Switch/3
  Data Store Read10/1 -> Divide1/2
  Data Store Read2/1 -> Add1/2, Divide1/1
  Divide/1 -> Add1/1
  Switch/1 -> Divide3/1, Data Store Write/1
  Add1/1 -> Switch/1
  Add/1 -> Switch/2, Divide/2, Divide/1  "fTemp"
  Abs/1 -> Add/1
  Data Store Read1/1 -> Add/2, Max/2
  Data Store Read/1 -> Abs/1

== system Target_Control_System/Target_Control_System/MainLoop/tiltMotor_mainLoop/mainTask_tilt/motorTaskMainFastStep(&oTilt)/Control Loops - Tilt/Flux Weakening Tilt ==
  Constant : Constant  Value=0  OutDataTypeStr=single  SampleTime=-1
  oRampDataIdRef_.fSetpoint : Outport
  wires:
  Constant/1 -> oRampDataIdRef_.fSetpoint/1
